simulink model "Gen_MPC"  (R2019b)
settings: Solver=VariableStepAuto  StartTime=0.0  StopTime=Time(end)  RelTol=1e-3
undefined symbols (not defined in the file): A, B
libraries: mpclib x2, cstblocks x2
settings Model: Creator=shouv  LastModifiedBy=shouv

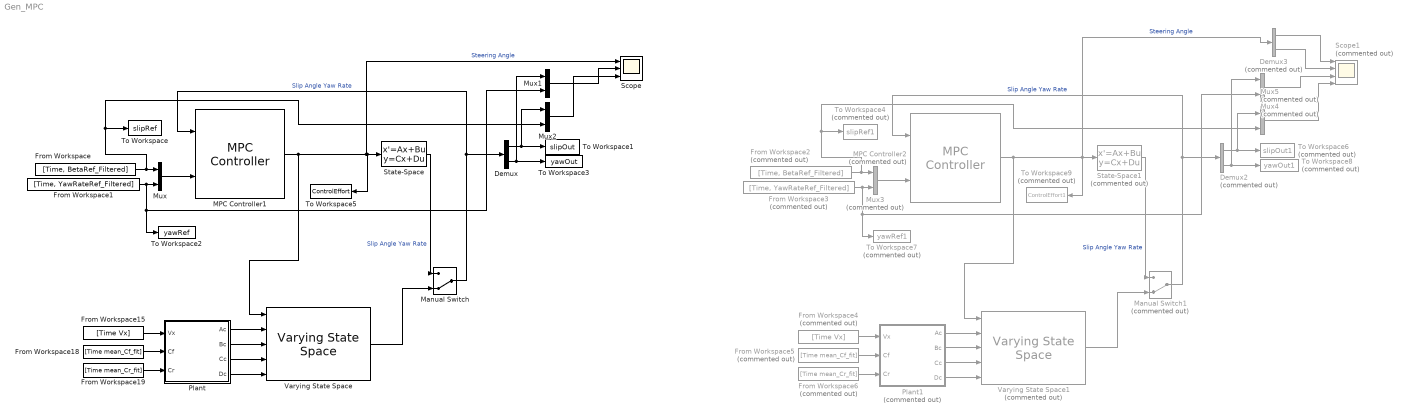
== system Gen_MPC ==
  Demux : Demux  Outputs=2
  Demux2 : Demux  Commented=on  Outputs=2
  Demux3 : Demux  Commented=on  Outputs=2
  From Workspace : FromWorkspace  VariableName=[Time, BetaRef_Filtered]  SampleTime=0
  From Workspace1 : FromWorkspace  VariableName=[Time, YawRateRef_Filtered]  SampleTime=0
  From Workspace15 : FromWorkspace  VariableName=[Time Vx]  SampleTime=0
  From Workspace18 : FromWorkspace  VariableName=[Time mean_Cf_fit]  SampleTime=0
  From Workspace19 : FromWorkspace  VariableName=[Time mean_Cr_fit]  SampleTime=0
  From Workspace2 : FromWorkspace  Commented=on  VariableName=[Time, BetaRef_Filtered]  SampleTime=0
  From Workspace3 : FromWorkspace  Commented=on  VariableName=[Time, YawRateRef_Filtered]  SampleTime=0
  From Workspace4 : FromWorkspace  Commented=on  VariableName=[Time Vx]  SampleTime=0
  From Workspace5 : FromWorkspace  Commented=on  VariableName=[Time mean_Cf_fit]  SampleTime=0
  From Workspace6 : FromWorkspace  Commented=on  VariableName=[Time mean_Cr_fit]  SampleTime=0
  MPC Controller1 : mpclib/MPC Controller  SCDEnableBlockLinearizationSpecification=on  mpcobj=mpc1  is_multiple=0  enable_value=0  return_u0=off  updateMPCinCallerWorkspace=on  md_inport=off  mv_inport=off  uref_inport=off  return_cost=off  return_mvseq=off  return_qpstatus=off  return_xseq=off  return_state=off  return_ovseq=off  state_inport=off  umin_inport=off  umax_inport=off  ymin_inport=off  ymax_inport=off  cc_inport=off  ywt_inport=off  uwt_inport=off  duwt_inport=off  rhoeps_inport=off  pm_inport=off  MaximumP=10  HorizonChoice=FixedHorizon  n_ts=0.025  n_p=15  n_mv=1  n_md=0  n_ud=0  n_mo=2  n_uo=0  BlockDataType=double  SampleTimeInherited=off  switch_inport=off
  MPC Controller2 : mpclib/MPC Controller  Commented=on  SCDEnableBlockLinearizationSpecification=on  mpcobj=mpcIntegratedControl  is_multiple=0  enable_value=0  return_u0=off  updateMPCinCallerWorkspace=on  md_inport=off  mv_inport=off  uref_inport=off  return_cost=off  return_mvseq=off  return_qpstatus=off  return_xseq=off  return_state=off  return_ovseq=off  state_inport=off  umin_inport=off  umax_inport=off  ymin_inport=off  ymax_inport=off  cc_inport=off  ywt_inport=off  uwt_inport=off  duwt_inport=off  rhoeps_inport=off  pm_inport=off  MaximumP=10  HorizonChoice=FixedHorizon  n_ts=0.025  n_p=3  n_mv=2  n_md=0  n_ud=0  n_mo=2  n_uo=0  BlockDataType=double  SampleTimeInherited=off  switch_inport=off
  Manual Switch : ManualSwitch  CurrentSetting=0
  Manual Switch1 : ManualSwitch  Commented=on  CurrentSetting=0
  Mux : Mux  Inputs=2
  Mux1 : Mux  Inputs=2
  Mux2 : Mux  Inputs=2
  Mux3 : Mux  Commented=on  Inputs=2
  Mux4 : Mux  Commented=on  Inputs=2
  Mux5 : Mux  Commented=on  Inputs=2
  Plant : MATLAB Function  TreatAsAtomicUnit=on
  Plant1 : MATLAB Function  Commented=on  TreatAsAtomicUnit=on
  Scope : Scope  NumInputPorts=3
  Scope1 : Scope  Commented=on  NumInputPorts=4
  State-Space : StateSpace  A=A  B=B  C=eye(2)  D=[0; 0]  InitialCondition=0
  State-Space1 : StateSpace  Commented=on  A=A  B=B  C=eye(2)  D=[0 0; 0 0]  InitialCondition=0
  To Workspace : ToWorkspace  VariableName=slipRef  SampleTime=-1
  To Workspace1 : ToWorkspace  VariableName=slipOut  SampleTime=-1
  To Workspace2 : ToWorkspace  VariableName=yawRef  SampleTime=-1
  To Workspace3 : ToWorkspace  VariableName=yawOut  SampleTime=-1
  To Workspace4 : ToWorkspace  Commented=on  VariableName=slipRef1  SampleTime=-1
  To Workspace5 : ToWorkspace  VariableName=ControlEffort  SampleTime=-1
  To Workspace6 : ToWorkspace  Commented=on  VariableName=slipOut1  SampleTime=-1
  To Workspace7 : ToWorkspace  Commented=on  VariableName=yawRef1  SampleTime=-1
  To Workspace8 : ToWorkspace  Commented=on  VariableName=yawOut1  SampleTime=-1
  To Workspace9 : ToWorkspace  Commented=on  VariableName=ControlEffort1  SampleTime=-1
  Varying State Space : cstblocks/Linear Parameter Varying/Varying State Space  x0=0  xNames=''  OutputX=off  OutputDX=off
      settings: SourceProductName=Control System Toolbox
  Varying State Space1 : cstblocks/Linear Parameter Varying/Varying State Space  Commented=on  x0=0  xNames=''  OutputX=off  OutputDX=off
      settings: SourceProductName=Control System Toolbox
  wires:
  From Workspace/1 -> Mux2/2, To Workspace/1, Mux/1
  Mux/1 -> MPC Controller1/2
  From Workspace1/1 -> Mux1/2, To Workspace2/1, Mux/2
  MPC Controller1/1 -> Scope/1, To Workspace5/1, State-Space/1, Varying State Space/1  "Steering Angle"
  Demux/2 -> Mux1/1, To Workspace3/1
  Demux/1 -> Mux2/1, To Workspace1/1
  Manual Switch/1 -> MPC Controller1/1, Demux/1  "Slip Angle Yaw Rate"
  Mux1/1 -> Scope/2
  Mux2/1 -> Scope/3
  From Workspace18/1 -> Plant/2(Cf)
  Plant/1(Ac) -> Varying State Space/2
  Plant/3(Cc) -> Varying State Space/4
  Plant/4(Dc) -> Varying State Space/5
  From Workspace15/1 -> Plant/1(Vx)
  Plant/2(Bc) -> Varying State Space/3
  From Workspace19/1 -> Plant/3(Cr)
  Varying State Space/1 -> Manual Switch/2
  State-Space/1 -> Manual Switch/1  "Slip Angle Yaw Rate"
  Manual Switch1/1 -> MPC Controller2/1, Demux2/1  "Slip Angle Yaw Rate"
  Varying State Space1/1 -> Manual Switch1/2
  Plant1/2(Bc) -> Varying State Space1/3
  From Workspace4/1 -> Plant1/1(Vx)
  Plant1/4(Dc) -> Varying State Space1/5
  Plant1/1(Ac) -> Varying State Space1/2
  From Workspace5/1 -> Plant1/2(Cf)
  Mux5/1 -> Scope1/4
  Demux2/1 -> Mux5/1, To Workspace6/1
  Mux4/1 -> Scope1/3
  Demux3/1 -> Scope1/1
  From Workspace6/1 -> Plant1/3(Cr)
  Mux3/1 -> MPC Controller2/2
  Demux3/2 -> Scope1/2
  Demux2/2 -> Mux4/1, To Workspace8/1
  MPC Controller2/1 -> Demux3/1, To Workspace9/1, State-Space1/1, Varying State Space1/1  "Steering Angle"
  From Workspace2/1 -> Mux5/2, To Workspace4/1, Mux3/1
  From Workspace3/1 -> Mux4/2, To Workspace7/1, Mux3/2
  State-Space1/1 -> Manual Switch1/1  "Slip Angle Yaw Rate"
  Plant1/3(Cc) -> Varying State Space1/4

== matlab function Gen_MPC/Plant ==
  data: Vx input; Ac output; Cf input; Cr input; Bc output; Cc output; Dc output
function [Ac, Bc, Cc, Dc]  = fcn(Vx,Cf,Cr)

% Model parameters
m = 1650;
Iz = 3234;
lf = 1.4;
lr = 1.65;

% Continuous-time model
Ac=[-(Cf+Cr)/(m*Vx), -1-(lf*Cf-lr*Cr)/(m*Vx^2);
    -(lf*Cf-lr*Cr)/Iz, -(lf^2*Cf+lr^2*Cr)/(Iz*Vx)];

Bc=[Cf/(m*Vx);(lf*Cf)/Iz];

Cc=eye(2);

Dc=zeros(2,1);

%dotX = Ac*x+Bc*steer;

== matlab function Gen_MPC/Plant1 ==
  data: Vx input; Ac output; Cf input; Cr input; Bc output; Cc output; Dc output
function [Ac, Bc, Cc, Dc]  = fcn(Vx,Cf,Cr)

% Model parameters
m = 1650;
Iz = 3234;
lf = 1.4;
lr = 1.65;

% Continuous-time model
Ac=[-(Cf+Cr)/(m*Vx), -1-(lf*Cf-lr*Cr)/(m*Vx^2);
    -(lf*Cf-lr*Cr)/Iz, -(lf^2*Cf+lr^2*Cr)/(Iz*Vx)];

Bc=[Cf/(m*Vx) 0;(lf*Cf)/Iz 1/Iz];

Cc=eye(2);

Dc=zeros(2,2);

%dotX = Ac*x+Bc*steer;
